simulink model "navcomb"  (R2025b)
settings: Solver=VariableStepAuto  StartTime=0.0  StopTime=10.0  RelTol=1e-3
values from neighbouring files (symbols this model uses):
  x0 = [0 ... (first row only)    [initialiseGEODETIC.m]
undefined symbols (not defined in the file or in its folder): RCAM_model_new
settings Model: Creator=smthejaswini  LastModifiedBy=smthejaswini

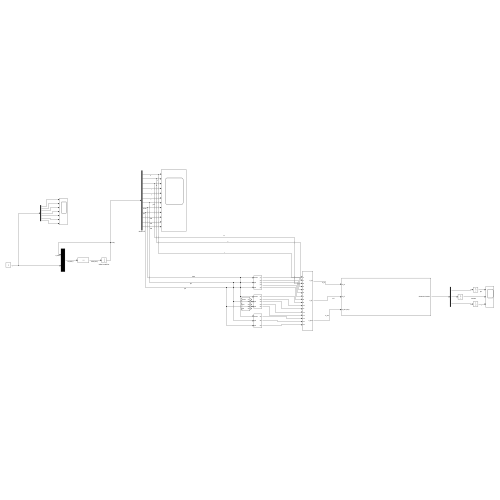
[thumbnail: Simulink's stored preview of the top-level diagram]
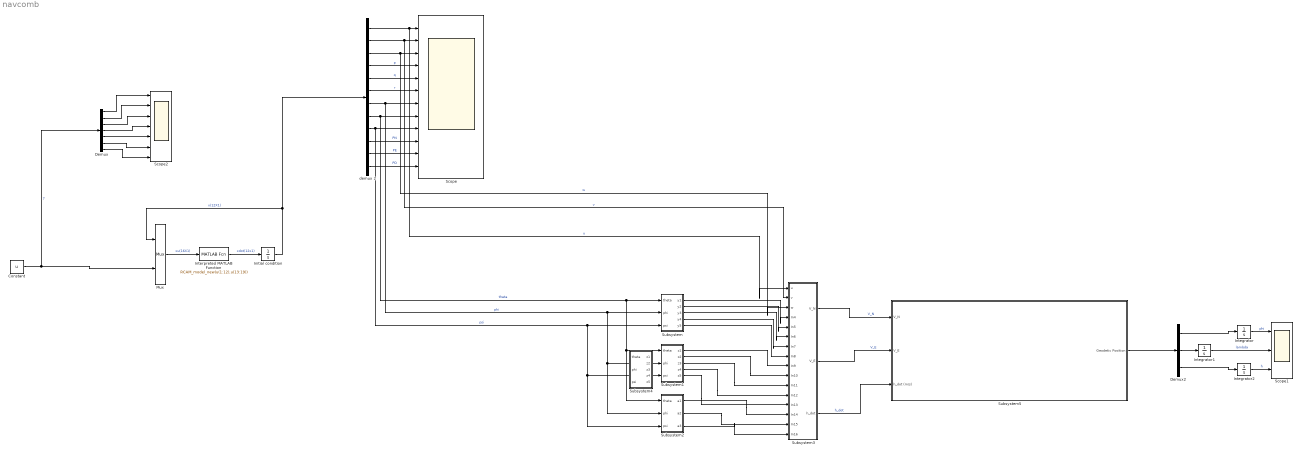
== system navcomb ==
  Constant : Constant  Value=u
  Demux : Demux  Outputs=7
  Demux2 : Demux  Outputs=3
  Initial condition : Integrator  InitialCondition=x0
  Integrator : Integrator
  Integrator1 : Integrator
  Integrator2 : Integrator
  Interpreted MATLAB Function : MATLABFcn  MATLABFcn=RCAM_model_new(u(1:12),u(13:19))
  Mux : Mux  Inputs=2
  Scope : Scope  NumInputPorts=12
  Scope1 : Scope  NumInputPorts=3
  Scope2 : Scope  NumInputPorts=7
      settings: DataLoggingVariableName=ScopeData2
  Subsystem : Subsystem
  Subsystem1 : Subsystem
  Subsystem2 : Subsystem
  Subsystem3 : Subsystem
  Subsystem4 : Subsystem
  Subsystem5 : Subsystem
  demux 2 : Demux  Outputs=12
  wires:
  Integrator2/1 -> Scope1/3  "h"
  Integrator/1 -> Scope1/1  "phi"
  Subsystem2/3(a3) -> Subsystem3/16(In16)
  Subsystem/1(y1) -> Subsystem3/4(In4)
  Subsystem/3(y3) -> Subsystem3/6(In6)
  demux 2/4 -> Scope/4  "p"
  demux 2/5 -> Scope/5  "q"
  Subsystem1/2(z2) -> Subsystem3/10(In10)
  demux 2/12 -> Scope/12  "PD"
  Demux2/3 -> Integrator2/1
  Subsystem3/3(h_dot) -> Subsystem5/3(h_dot (m/s))  "h_dot"
  Subsystem3/1(V_N) -> Subsystem5/1(V_N)  "V_N"
  Subsystem5/1("Geodetic Position ") -> Demux2/1
  Subsystem1/5(z5) -> Subsystem3/13(In13)
  Subsystem1/3(z3) -> Subsystem3/11(In11)
  Subsystem/2(y2) -> Subsystem3/5(In5)
  demux 2/10 -> Scope/10  "PN"
  Demux2/2 -> Integrator1/1
  demux 2/11 -> Scope/11  "PE"
  Integrator1/1 -> Scope1/2  "lambda"
  demux 2/6 -> Scope/6  "r"
  Subsystem3/2(V_E) -> Subsystem5/2(V_E)  "V_E"
  demux 2/9 -> Subsystem2/3(psi), Subsystem1/3(psi), Subsystem/3(psi), Scope/9  "psi"
  Subsystem/4(y4) -> Subsystem3/7(In7)
  Subsystem1/4(z4) -> Subsystem3/12(In12)
  demux 2/2 -> Subsystem3/2(v), Scope/2  "v"
  Subsystem2/2(a2) -> Subsystem3/15(In15)
  Subsystem/5(y5) -> Subsystem3/8(In8)
  Demux2/1 -> Integrator/1
  demux 2/7 -> Subsystem2/2(phi), Subsystem1/2(phi), Subsystem/2(phi), Scope/7  "phi"
  demux 2/1 -> Subsystem3/1(u), Scope/1  "u"
  demux 2/3 -> Subsystem3/3(w), Scope/3  "w"
  Subsystem1/1(z1) -> Subsystem3/9(In9)
  demux 2/8 -> Subsystem2/1(theta), Subsystem1/1(theta), Subsystem/1(theta), Scope/8  "theta"
  Subsystem2/1(a1) -> Subsystem3/14(In14)
  Demux/1 -> Scope2/1
  Demux/2 -> Scope2/2
  Demux/5 -> Scope2/5
  Demux/6 -> Scope2/6
  Demux/7 -> Scope2/7
  Demux/3 -> Scope2/3
  Demux/4 -> Scope2/4
  Mux/1 -> Interpreted MATLAB Function/1  "xu(16X1)"
  Initial condition/1 -> demux 2/1, Mux/1  "x(12X1)"
  Interpreted MATLAB Function/1 -> Initial condition/1  "xdot(12x1)"
  Constant/1 -> Demux/1, Mux/2  "7"

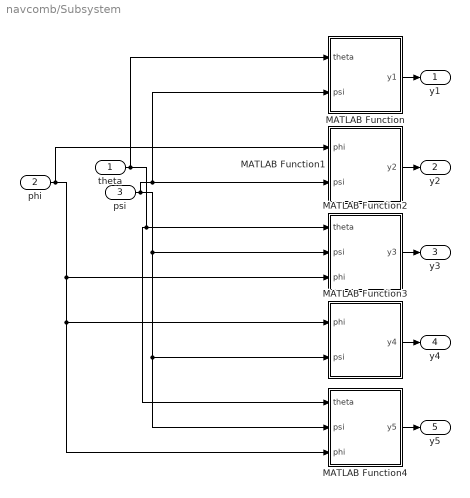
== system navcomb/Subsystem ==
  theta : Inport
  phi : Inport  Port=2
  psi : Inport  Port=3
  MATLAB Function : MATLAB Function  TreatAsAtomicUnit=on
  MATLAB Function1 : MATLAB Function  TreatAsAtomicUnit=on
  MATLAB Function2 : MATLAB Function  TreatAsAtomicUnit=on
  MATLAB Function3 : MATLAB Function  TreatAsAtomicUnit=on
  MATLAB Function4 : MATLAB Function  TreatAsAtomicUnit=on
  y1 : Outport
  y2 : Outport  Port=2
  y3 : Outport  Port=3
  y4 : Outport  Port=4
  y5 : Outport  Port=5
  wires:
  MATLAB Function4/1(y5) -> y5/1
  MATLAB Function3/1(y4) -> y4/1
  psi/1 -> MATLAB Function4/2(psi), MATLAB Function3/2(psi), MATLAB Function2/2(psi), MATLAB Function1/2(psi), MATLAB Function/2(psi)
  phi/1 -> MATLAB Function4/3(phi), MATLAB Function3/1(phi), MATLAB Function2/3(phi), MATLAB Function1/1(phi)
  MATLAB Function1/1(y2) -> y2/1
  theta/1 -> MATLAB Function4/1(theta), MATLAB Function2/1(theta), MATLAB Function/1(theta)
  MATLAB Function/1(y1) -> y1/1
  MATLAB Function2/1(y3) -> y3/1

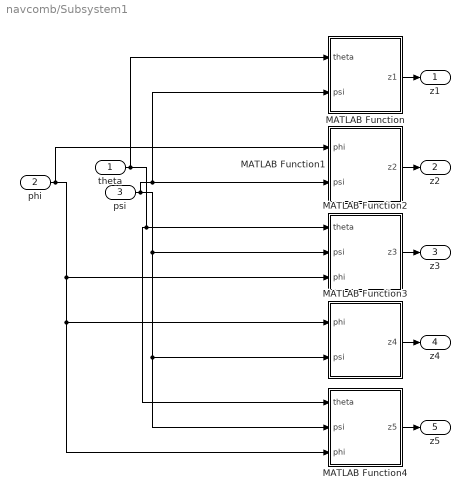
== system navcomb/Subsystem1 ==
  theta : Inport
  phi : Inport  Port=2
  psi : Inport  Port=3
  MATLAB Function : MATLAB Function  TreatAsAtomicUnit=on
  MATLAB Function1 : MATLAB Function  TreatAsAtomicUnit=on
  MATLAB Function2 : MATLAB Function  TreatAsAtomicUnit=on
  MATLAB Function3 : MATLAB Function  TreatAsAtomicUnit=on
  MATLAB Function4 : MATLAB Function  TreatAsAtomicUnit=on
  z1 : Outport
  z2 : Outport  Port=2
  z3 : Outport  Port=3
  z4 : Outport  Port=4
  z5 : Outport  Port=5
  wires:
  MATLAB Function4/1(z5) -> z5/1
  MATLAB Function3/1(z4) -> z4/1
  psi/1 -> MATLAB Function4/2(psi), MATLAB Function3/2(psi), MATLAB Function2/2(psi), MATLAB Function1/2(psi), MATLAB Function/2(psi)
  phi/1 -> MATLAB Function4/3(phi), MATLAB Function3/1(phi), MATLAB Function2/3(phi), MATLAB Function1/1(phi)
  MATLAB Function1/1(z2) -> z2/1
  theta/1 -> MATLAB Function4/1(theta), MATLAB Function2/1(theta), MATLAB Function/1(theta)
  MATLAB Function/1(z1) -> z1/1
  MATLAB Function2/1(z3) -> z3/1

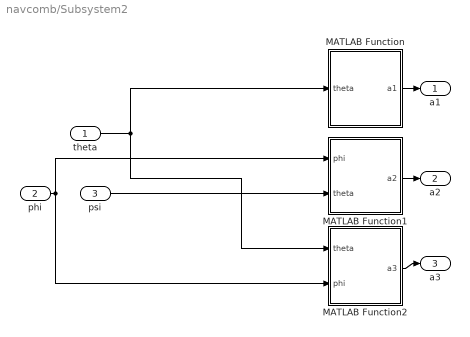
== system navcomb/Subsystem2 ==
  theta : Inport
  phi : Inport  Port=2
  psi : Inport  Port=3
  MATLAB Function : MATLAB Function  TreatAsAtomicUnit=on
  MATLAB Function1 : MATLAB Function  TreatAsAtomicUnit=on
  MATLAB Function2 : MATLAB Function  TreatAsAtomicUnit=on
  a1 : Outport
  a2 : Outport  Port=2
  a3 : Outport  Port=3
  wires:
  psi/1 -> MATLAB Function1/2(theta)
  phi/1 -> MATLAB Function2/2(phi), MATLAB Function1/1(phi)
  MATLAB Function1/1(a2) -> a2/1
  theta/1 -> MATLAB Function2/1(theta), MATLAB Function/1(theta)
  MATLAB Function/1(a1) -> a1/1
  MATLAB Function2/1(a3) -> a3/1

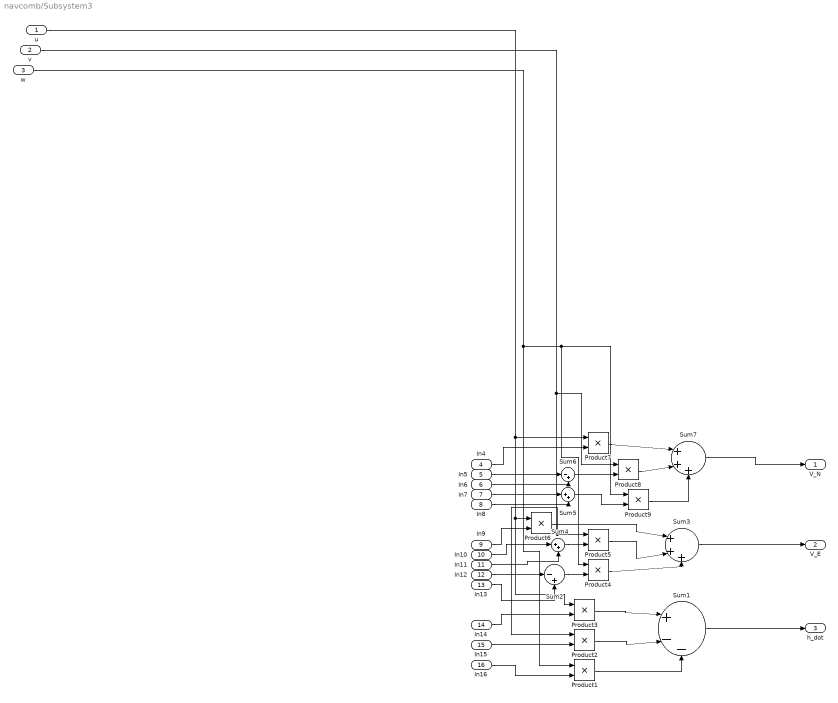
== system navcomb/Subsystem3 ==
  u : Inport
  v : Inport  Port=2
  w : Inport  Port=3
  In4 : Inport  Port=4
  In5 : Inport  Port=5
  In6 : Inport  Port=6
  In7 : Inport  Port=7
  In8 : Inport  Port=8
  In9 : Inport  Port=9
  In10 : Inport  Port=10
  In11 : Inport  Port=11
  In12 : Inport  Port=12
  In13 : Inport  Port=13
  In14 : Inport  Port=14
  In15 : Inport  Port=15
  In16 : Inport  Port=16
  Product{1..9} (9 alike) : Product
  Sum1 : Sum  Inputs=|+--
  Sum2 : Sum  Inputs=|-+
  Sum3 : Sum  Inputs=|+++
  Sum4 : Sum  Inputs=|++
  Sum5 : Sum  Inputs=|++
  Sum6 : Sum  Inputs=|-+
  Sum7 : Sum  Inputs=|+++
  V_N : Outport
  V_E : Outport  Port=2
  h_dot : Outport  Port=3
  wires:
  u/1 -> Product3/1, Product6/1, Product7/1
  Product3/1 -> Sum1/1
  In5/1 -> Sum6/1
  In13/1 -> Sum2/2
  Product5/1 -> Sum3/2
  Sum1/1 -> h_dot/1
  v/1 -> Product2/1, Product5/1, Product8/1
  w/1 -> Product1/1, Product4/1, Product9/1
  Sum6/1 -> Product8/2
  In6/1 -> Sum6/2
  In11/1 -> Sum4/2
  Product9/1 -> Sum7/3
  Sum2/1 -> Product4/2
  Product1/1 -> Sum1/3
  Product4/1 -> Sum3/3
  Sum4/1 -> Product5/2
  Product6/1 -> Sum3/1
  Product8/1 -> Sum7/2
  Product7/1 -> Sum7/1
  Sum5/1 -> Product9/2
  In4/1 -> Product7/2
  Product2/1 -> Sum1/2
  In7/1 -> Sum5/1
  In8/1 -> Sum5/2
  Sum7/1 -> V_N/1
  In10/1 -> Sum4/1
  Sum3/1 -> V_E/1
  In9/1 -> Product6/2
  In14/1 -> Product3/2
  In12/1 -> Sum2/1
  In16/1 -> Product1/2
  In15/1 -> Product2/2

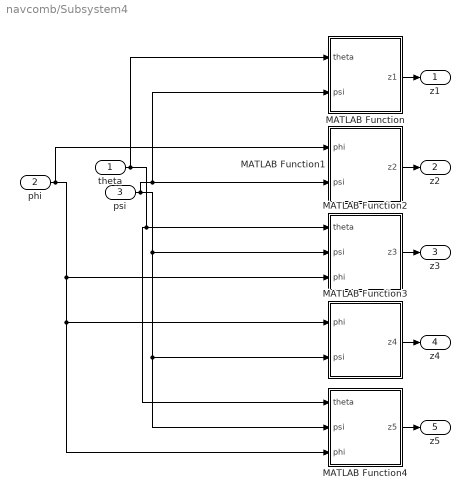
== system navcomb/Subsystem4 ==
  theta : Inport
  phi : Inport  Port=2
  psi : Inport  Port=3
  MATLAB Function : MATLAB Function  TreatAsAtomicUnit=on
  MATLAB Function1 : MATLAB Function  TreatAsAtomicUnit=on
  MATLAB Function2 : MATLAB Function  TreatAsAtomicUnit=on
  MATLAB Function3 : MATLAB Function  TreatAsAtomicUnit=on
  MATLAB Function4 : MATLAB Function  TreatAsAtomicUnit=on
  z1 : Outport
  z2 : Outport  Port=2
  z3 : Outport  Port=3
  z4 : Outport  Port=4
  z5 : Outport  Port=5
  wires:
  MATLAB Function2/1(z3) -> z3/1
  MATLAB Function/1(z1) -> z1/1
  theta/1 -> MATLAB Function/1(theta), MATLAB Function2/1(theta), MATLAB Function4/1(theta)
  MATLAB Function1/1(z2) -> z2/1
  phi/1 -> MATLAB Function1/1(phi), MATLAB Function2/3(phi), MATLAB Function3/1(phi), MATLAB Function4/3(phi)
  psi/1 -> MATLAB Function/2(psi), MATLAB Function1/2(psi), MATLAB Function2/2(psi), MATLAB Function3/2(psi), MATLAB Function4/2(psi)
  MATLAB Function3/1(z4) -> z4/1
  MATLAB Function4/1(z5) -> z5/1

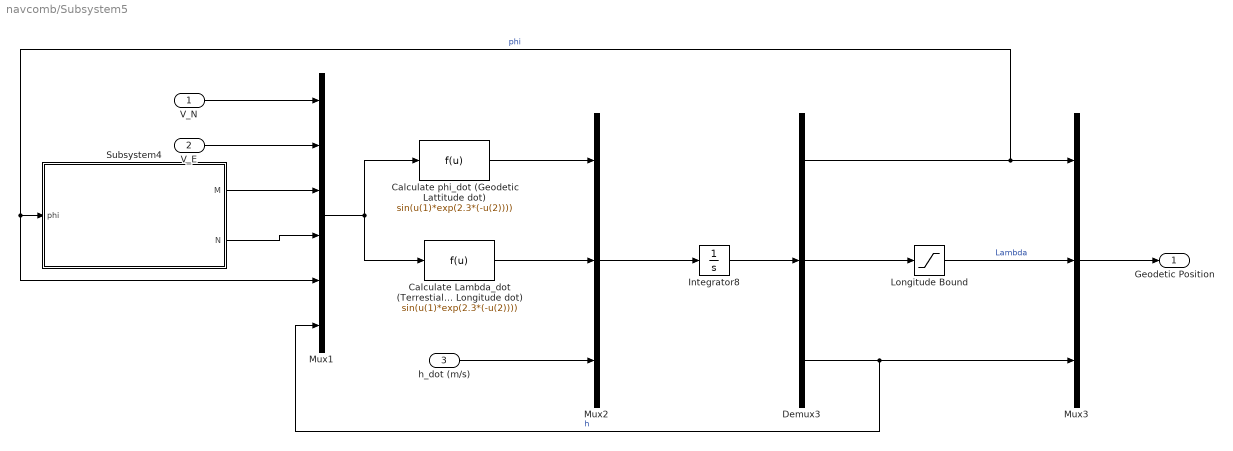
== system navcomb/Subsystem5 ==
  V_N : Inport
  V_E : Inport  Port=2
  h_dot (m/s) : Inport  Port=3
  Calculate Lambda_dot (Terrestial Longitude dot) : Fcn  Expr=sin(u(1)*exp(2.3*(-u(2))))
  "Calculate phi_dot (Geodetic Lattitude dot) " : Fcn  Expr=sin(u(1)*exp(2.3*(-u(2))))
  Demux3 : Demux  Outputs=3
  Integrator8 : Integrator
  "Longitude Bound " : Saturate  UpperLimit=pi  LowerLimit=-pi
  Mux1 : Mux  Inputs=6
  Mux2 : Mux  Inputs=3
  Mux3 : Mux  Inputs=3
  Subsystem4 : Subsystem
  "Geodetic Position " : Outport
  wires:
  Demux3/1 -> Mux1/5, Subsystem4/1(phi), Mux3/1  "phi"
  Calculate Lambda_dot (Terrestial Longitude dot)/1 -> Mux2/2
  "Calculate phi_dot (Geodetic Lattitude dot) "/1 -> Mux2/1
  h_dot (m/s)/1 -> Mux2/3
  Demux3/2 -> "Longitude Bound "/1
  Mux2/1 -> Integrator8/1
  Mux3/1 -> "Geodetic Position "/1
  Subsystem4/2(N) -> Mux1/4
  Subsystem4/1(M) -> Mux1/3
  "Longitude Bound "/1 -> Mux3/2  "Lambda"
  Integrator8/1 -> Demux3/1
  Demux3/3 -> Mux1/6, Mux3/3  "h"
  V_E/1 -> Mux1/2
  V_N/1 -> Mux1/1
  Mux1/1 -> Calculate Lambda_dot (Terrestial Longitude dot)/1, "Calculate phi_dot (Geodetic Lattitude dot) "/1

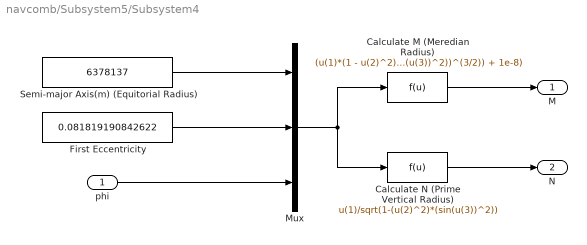
== system navcomb/Subsystem5/Subsystem4 ==
  phi : Inport
  "Calculate M (Meredian Radius) " : Fcn  Expr=(u(1)*(1 - u(2)^2)) / ((((1 - u(2)^2) * (sin(u(3))^2))^(3/2)) + 1e-8)
  Calculate N (Prime Vertical Radius) : Fcn  Expr=u(1)/sqrt(1-(u(2)^2)*(sin(u(3))^2))
  First Eccentricity : Constant  Value=0.081819190842622
  Mux : Mux  Inputs=3
  Semi-major Axis(m) (Equitorial Radius) : Constant  Value=6378137
  M : Outport
  N : Outport  Port=2
  wires:
  First Eccentricity/1 -> Mux/2
  phi/1 -> Mux/3
  Calculate N (Prime Vertical Radius)/1 -> N/1
  Mux/1 -> Calculate N (Prime Vertical Radius)/1, "Calculate M (Meredian Radius) "/1
  "Calculate M (Meredian Radius) "/1 -> M/1
  Semi-major Axis(m) (Equitorial Radius)/1 -> Mux/1

== matlab function navcomb/Subsystem2/MATLAB Function1 ==
  data: phi input; a2 output; theta input
function a2 = fcn(phi,theta)

a2 = sin(phi)*cos(theta);

== matlab function navcomb/Subsystem2/MATLAB Function2 ==
  data: theta input; a3 output; phi input
function a3 = fcn(theta,phi)

a3 = cos(phi)*cos(theta);

== matlab function navcomb/Subsystem4/MATLAB Function ==
  data: theta input; z1 output; psi input
function z1 = fcn(theta,psi)

z1 = cos(theta)*sin(psi);

== matlab function navcomb/Subsystem4/MATLAB Function1 ==
  data: phi input; z2 output; psi input
function z2 = fcn(phi,psi)

z2 = cos(phi)*cos(psi);

== matlab function navcomb/Subsystem4/MATLAB Function2 ==
  data: theta input; z3 output; psi input; phi input
function z3 = fcn(theta,psi,phi)

z3 = sin(phi)*sin(theta)*sin(psi);

== matlab function navcomb/Subsystem4/MATLAB Function3 ==
  data: phi input; z4 output; psi input
function z4 = fcn(phi,psi)

z4 = sin(phi)*cos(psi);

== matlab function navcomb/Subsystem4/MATLAB Function4 ==
  data: theta input; z5 output; psi input; phi input
function z5 = fcn(theta,psi,phi)

z5 = cos(phi)*sin(theta)*sin(psi);

== matlab function navcomb/Subsystem/MATLAB Function ==
  data: theta input; y1 output; psi input
function y1 = fcn(theta,psi)

y1 = cos(theta)*cos(psi);

== matlab function navcomb/Subsystem/MATLAB Function2 ==
  data: theta input; y3 output; psi input; phi input
function y3 = fcn(theta,psi,phi)

y3 = sin(phi)*sin(theta)*cos(psi);

== matlab function navcomb/Subsystem/MATLAB Function3 ==
  data: phi input; y4 output; psi input
function y4 = fcn(phi,psi)

y4 = sin(phi)*sin(psi);

== matlab function navcomb/Subsystem/MATLAB Function4 ==
  data: theta input; y5 output; psi input; phi input
function y5 = fcn(theta,psi,phi)

y5 = cos(phi)*sin(theta)*cos(psi);

== matlab function navcomb/Subsystem1/MATLAB Function ==
  data: theta input; z1 output; psi input
function z1 = fcn(theta,psi)

z1 = cos(theta)*sin(psi);

== matlab function navcomb/Subsystem1/MATLAB Function1 ==
  data: phi input; z2 output; psi input
function z2 = fcn(phi,psi)

z2 = cos(phi)*cos(psi);

== matlab function navcomb/Subsystem1/MATLAB Function2 ==
  data: theta input; z3 output; psi input; phi input
function z3 = fcn(theta,psi,phi)

z3 = sin(phi)*sin(theta)*sin(psi);

== matlab function navcomb/Subsystem1/MATLAB Function3 ==
  data: phi input; z4 output; psi input
function z4 = fcn(phi,psi)

z4 = sin(phi)*cos(psi);

== matlab function navcomb/Subsystem1/MATLAB Function4 ==
  data: theta input; z5 output; psi input; phi input
function z5 = fcn(theta,psi,phi)

z5 = cos(phi)*sin(theta)*sin(psi);

== matlab function navcomb/Subsystem/MATLAB Function1 ==
  data: phi input; y2 output; psi input
function y2 = fcn(phi,psi)

y2 = cos(phi)*sin(psi);

== matlab function navcomb/Subsystem2/MATLAB Function ==
  data: theta input; a1 output
function a1 = fcn(theta)

a1 = sin(theta);
